simulink subsystem "s4EMSSC"  (R2024b)
settings: Solver=VariableStepAuto  StartTime=0.0  StopTime=10.0  RelTol=1e-3
undefined symbols (not defined in the file): EM1, EM2, EM3, EM4, HVDCNeg, HVDCPos, ThrmEM1, ThrmEM2, ThrmEM3, ThrmEM4
libraries: fl_lib x28, nesl_utility_internal x20
settings Model: ModifiedByFormat=The MathWorks, Inc.  Creator=The MathWorks, Inc.  LastModifiedBy=The MathWorks, Inc.
settings RTWCC: GPUComputeCapability=3.5

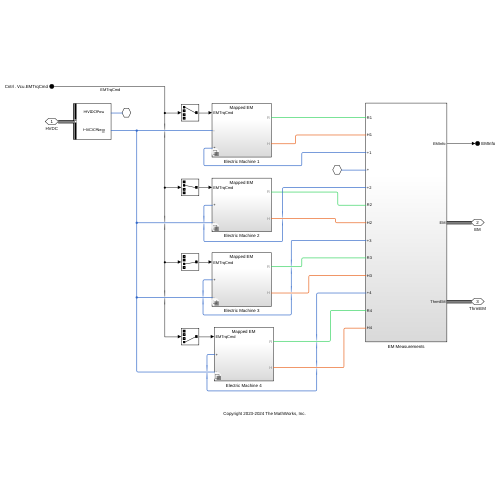
[thumbnail: Simulink's stored preview of the top-level diagram]
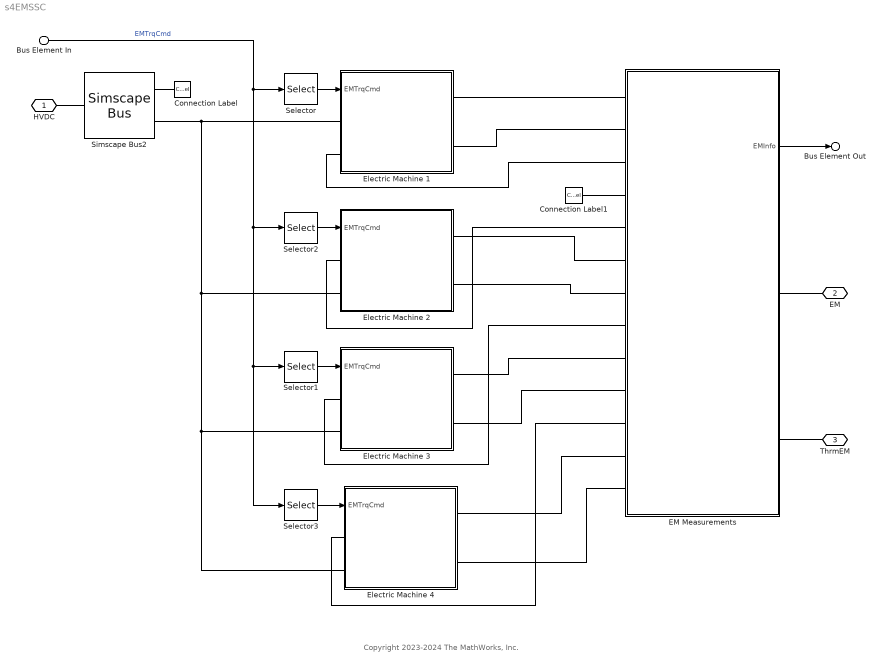
== system s4EMSSC ==
  note: Copyright 2023-2024 The MathWorks, Inc.
  Bus Element In : Inport  PortName=Cntrl  Element=Vcu.EMTrqCmd
  Connection Label : ConnectionLabel  Label=HVDCPos
  Connection Label1 : ConnectionLabel  Label=HVDCPos
  EM Measurements : Subsystem
  Electric Machine 1 : Subsystem  Variant=on  VariantControlMode=label  LabelModeActiveChoice=Mapped EM
  Electric Machine 2 : Subsystem  Variant=on  VariantControlMode=label  LabelModeActiveChoice=Mapped EM
  Electric Machine 3 : Subsystem  Variant=on  VariantControlMode=label  LabelModeActiveChoice=Mapped EM
  Electric Machine 4 : Subsystem  Variant=on  VariantControlMode=label  LabelModeActiveChoice=Mapped EM
  Selector : Selector  InputPortWidth=4  IndexOptions=Index vector (dialog)  Indices=[1]  OutputSizes=1
  Selector1 : Selector  InputPortWidth=4  IndexOptions=Index vector (dialog)  Indices=[3]  OutputSizes=1
  Selector2 : Selector  InputPortWidth=4  IndexOptions=Index vector (dialog)  Indices=[2]  OutputSizes=1
  Selector3 : Selector  InputPortWidth=4  IndexOptions=Index vector (dialog)  Indices=[4]  OutputSizes=1
  Simscape Bus2 : SimscapeBus  HierarchyStrings=HVDCPos;HVDCNeg
  HVDC : PMIOPort  Side=Left
  EM : PMIOPort  Port=2  Side=Right
  ThrmEM : PMIOPort  Port=3  Side=Right
  Bus Element Out : Outport  PortName=EMInfo
  wires:
  Selector3/1 -> Electric Machine 4/1(EMTrqCmd)
  Bus Element In/1 -> Selector2/1, Selector1/1, Selector3/1, Selector/1  "EMTrqCmd"
  Selector2/1 -> Electric Machine 2/1(EMTrqCmd)
  Selector/1 -> Electric Machine 1/1(EMTrqCmd)
  Selector1/1 -> Electric Machine 3/1(EMTrqCmd)
  EM Measurements/1(EMInfo) -> Bus Element Out/1
  connections:
  Simscape Bus2/LConn2 -- Electric Machine 3/LConn2 -- Electric Machine 4/LConn2 -- Electric Machine 2/LConn2 -- Electric Machine 1/LConn1
  HVDC/RConn1 -- Simscape Bus2/RConn1
  ThrmEM/RConn1 -- EM Measurements/RConn2
  EM Measurements/LConn9 -- Electric Machine 3/RConn1
  EM Measurements/LConn2 -- Electric Machine 1/RConn2
  EM Measurements/RConn1 -- EM/RConn1
  Electric Machine 2/RConn1 -- EM Measurements/LConn6
  Electric Machine 2/RConn2 -- EM Measurements/LConn7
  Electric Machine 1/RConn1 -- EM Measurements/LConn1
  EM Measurements/LConn5 -- Electric Machine 2/LConn1
  Connection Label1/LConn1 -- EM Measurements/LConn4
  Connection Label/LConn1 -- Simscape Bus2/LConn1
  EM Measurements/LConn3 -- Electric Machine 1/LConn2
  Electric Machine 3/LConn1 -- EM Measurements/LConn8
  Electric Machine 3/RConn2 -- EM Measurements/LConn10
  Electric Machine 4/LConn1 -- EM Measurements/LConn11
  Electric Machine 4/RConn1 -- EM Measurements/LConn12
  Electric Machine 4/RConn2 -- EM Measurements/LConn13

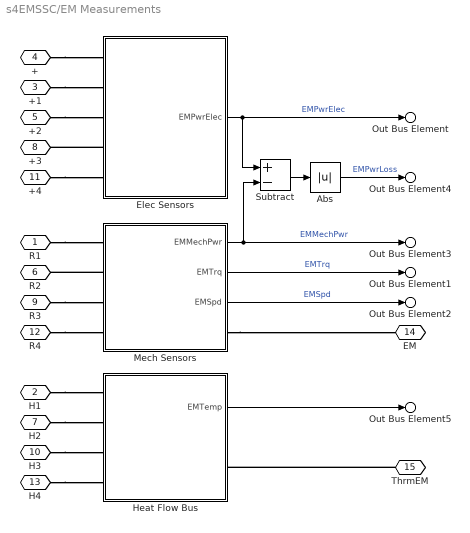
== system s4EMSSC/EM Measurements ==
  Abs : Abs  SaturateOnIntegerOverflow=off
  Elec Sensors : Subsystem
  Heat Flow Bus : Subsystem
  Mech Sensors : Subsystem
  Subtract : Sum  Inputs=+-
  R1 : PMIOPort  Side=Left
  H1 : PMIOPort  Port=2  Side=Left
  +1 : PMIOPort  Port=3  Side=Left
  + : PMIOPort  Port=4  Side=Left
  +2 : PMIOPort  Port=5  Side=Left
  R2 : PMIOPort  Port=6  Side=Left
  H2 : PMIOPort  Port=7  Side=Left
  +3 : PMIOPort  Port=8  Side=Left
  R3 : PMIOPort  Port=9  Side=Left
  H3 : PMIOPort  Port=10  Side=Left
  +4 : PMIOPort  Port=11  Side=Left
  R4 : PMIOPort  Port=12  Side=Left
  H4 : PMIOPort  Port=13  Side=Left
  EM : PMIOPort  Port=14  Side=Right
  ThrmEM : PMIOPort  Port=15  Side=Right
  Out Bus Element : Outport  PortName=EMInfo  Element=EMPwrElec
  Out Bus Element1 : Outport  PortName=EMInfo  Element=EMTrq
  Out Bus Element2 : Outport  PortName=EMInfo  Element=EMSpd
  Out Bus Element3 : Outport  PortName=EMInfo  Element=EMMechPwr
  Out Bus Element4 : Outport  PortName=EMInfo  Element=EMPwrLoss
  Out Bus Element5 : Outport  PortName=EMInfo  Element=EMTemp
  wires:
  Mech Sensors/1(EMMechPwr) -> Subtract/2, Out Bus Element3/1  "EMMechPwr"
  Mech Sensors/3(EMSpd) -> Out Bus Element2/1  "EMSpd"
  Mech Sensors/2(EMTrq) -> Out Bus Element1/1  "EMTrq"
  Elec Sensors/1(EMPwrElec) -> Subtract/1, Out Bus Element/1  "EMPwrElec"
  Abs/1 -> Out Bus Element4/1  "EMPwrLoss"
  Subtract/1 -> Abs/1
  Heat Flow Bus/1(EMTemp) -> Out Bus Element5/1
  connections:
  +4/RConn1 -- Elec Sensors/LConn5
  R4/RConn1 -- Mech Sensors/LConn4
  Elec Sensors/LConn4 -- +3/RConn1
  R3/RConn1 -- Mech Sensors/LConn3
  +2/RConn1 -- Elec Sensors/LConn3
  Mech Sensors/LConn2 -- R2/RConn1
  +1/RConn1 -- Elec Sensors/LConn2
  +/RConn1 -- Elec Sensors/LConn1
  R1/RConn1 -- Mech Sensors/LConn1
  ThrmEM/RConn1 -- Heat Flow Bus/RConn1
  Mech Sensors/RConn1 -- EM/RConn1
  H1/RConn1 -- Heat Flow Bus/LConn1
  H2/RConn1 -- Heat Flow Bus/LConn2
  H3/RConn1 -- Heat Flow Bus/LConn3
  H4/RConn1 -- Heat Flow Bus/LConn4

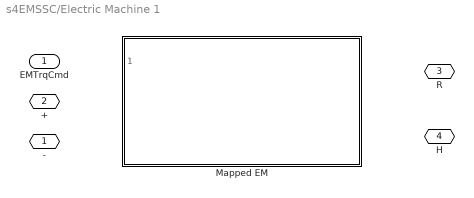
== system s4EMSSC/Electric Machine 1 ==
  EMTrqCmd : Inport
  Mapped EM : Subsystem  VariantControl=Mapped EM  ReferencedSubsystem=ElectricMachine1SSC
  - : PMIOPort  Side=Left
  + : PMIOPort  Port=2  Side=Left
  R : PMIOPort  Port=3  Side=Right
  H : PMIOPort  Port=4  Side=Right

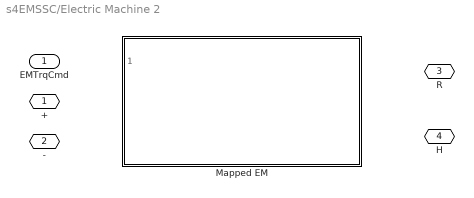
== system s4EMSSC/Electric Machine 2 ==
  EMTrqCmd : Inport
  Mapped EM : Subsystem  VariantControl=Mapped EM  ReferencedSubsystem=ElectricMachine2SSC
  + : PMIOPort  Side=Left
  - : PMIOPort  Port=2  Side=Left
  R : PMIOPort  Port=3  Side=Right
  H : PMIOPort  Port=4  Side=Right

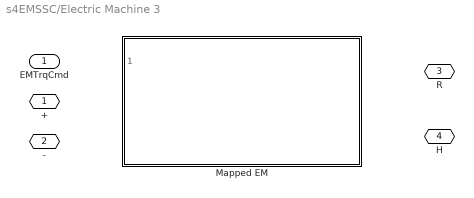
== system s4EMSSC/Electric Machine 3 ==
  EMTrqCmd : Inport
  Mapped EM : Subsystem  VariantControl=Mapped EM  ReferencedSubsystem=ElectricMachine3SSC
  + : PMIOPort  Side=Left
  - : PMIOPort  Port=2  Side=Left
  R : PMIOPort  Port=3  Side=Right
  H : PMIOPort  Port=4  Side=Right

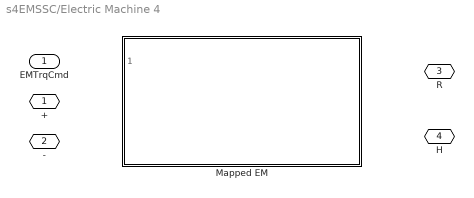
== system s4EMSSC/Electric Machine 4 ==
  EMTrqCmd : Inport
  Mapped EM : Subsystem  VariantControl=Mapped EM  ReferencedSubsystem=ElectricMachine4SSC
  + : PMIOPort  Side=Left
  - : PMIOPort  Port=2  Side=Left
  R : PMIOPort  Port=3  Side=Right
  H : PMIOPort  Port=4  Side=Right

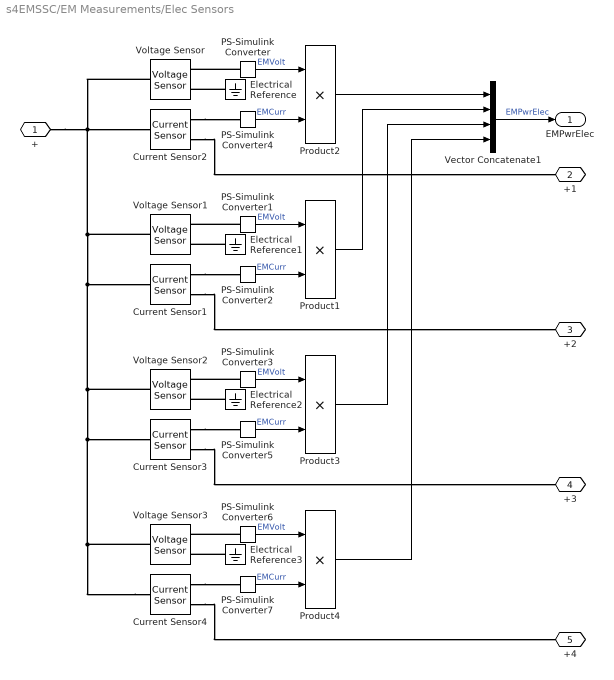
== system s4EMSSC/EM Measurements/Elec Sensors ==
  Current Sensor{1..4} (4 alike) : fl_lib/Electrical/Electrical Sensors/Current Sensor
  Electrical Reference{,1..3} (4 alike) : fl_lib/Electrical/Electrical Elements/Electrical Reference
  PS-Simulink Converter{,1,3,6} (4 alike) : nesl_utility_internal/PS-Simulink Converter  PhysicalDomain=network_engine_domain  SubClassName=ps_output  LeftPortType=input  RightPortType=output  PseudoPeriodic=off  Frequencies=[]  VectorFormat=1-D array  Unit=inherit  AffineConversion=off
  PS-Simulink Converter{2,4..5,7} (4 alike) : nesl_utility_internal/PS-Simulink Converter  PhysicalDomain=network_engine_domain  SubClassName=ps_output  LeftPortType=input  RightPortType=output  PseudoPeriodic=off  Frequencies=[]  VectorFormat=1-D array  Unit=1  AffineConversion=off
  Product{1..4} (4 alike) : Product
  Vector Concatenate1 : Concatenate  NumInputs=4
  Voltage Sensor{,1..3} (4 alike) : fl_lib/Electrical/Electrical Sensors/Voltage Sensor
  + : PMIOPort  Side=Left
  +1 : PMIOPort  Port=2  Side=Left
  +2 : PMIOPort  Port=3  Side=Left
  +3 : PMIOPort  Port=4  Side=Left
  +4 : PMIOPort  Port=5  Side=Left
  EMPwrElec : Outport
  wires:
  Product4/1 -> Vector Concatenate1/4
  PS-Simulink Converter7/1 -> Product4/2  "EMCurr"
  PS-Simulink Converter6/1 -> Product4/1  "EMVolt"
  PS-Simulink Converter3/1 -> Product3/1  "EMVolt"
  PS-Simulink Converter5/1 -> Product3/2  "EMCurr"
  Product3/1 -> Vector Concatenate1/3
  Product1/1 -> Vector Concatenate1/2
  Vector Concatenate1/1 -> EMPwrElec/1  "EMPwrElec"
  Product2/1 -> Vector Concatenate1/1
  PS-Simulink Converter2/1 -> Product1/2  "EMCurr"
  PS-Simulink Converter1/1 -> Product1/1  "EMVolt"
  PS-Simulink Converter/1 -> Product2/1  "EMVolt"
  PS-Simulink Converter4/1 -> Product2/2  "EMCurr"
  connections:
  Current Sensor4/RConn1 -- PS-Simulink Converter7/LConn1
  Current Sensor4/RConn2 -- +4/RConn1
  Electrical Reference3/LConn1 -- Voltage Sensor3/RConn2
  PS-Simulink Converter6/LConn1 -- Voltage Sensor3/RConn1
  PS-Simulink Converter3/LConn1 -- Voltage Sensor2/RConn1
  Electrical Reference2/LConn1 -- Voltage Sensor2/RConn2
  Current Sensor3/RConn2 -- +3/RConn1
  Current Sensor3/RConn1 -- PS-Simulink Converter5/LConn1
  Electrical Reference1/LConn1 -- Voltage Sensor1/RConn2
  Current Sensor1/RConn1 -- PS-Simulink Converter2/LConn1
  Current Sensor1/RConn2 -- +2/RConn1
  PS-Simulink Converter1/LConn1 -- Voltage Sensor1/RConn1
  PS-Simulink Converter/LConn1 -- Voltage Sensor/RConn1
  Electrical Reference/LConn1 -- Voltage Sensor/RConn2
  Current Sensor4/LConn1 -- Voltage Sensor3/LConn1 -- Voltage Sensor2/LConn1 -- Current Sensor2/LConn1 -- +/RConn1 -- Voltage Sensor/LConn1 -- Voltage Sensor1/LConn1 -- Current Sensor1/LConn1 -- Current Sensor3/LConn1
  Current Sensor2/RConn2 -- +1/RConn1
  Current Sensor2/RConn1 -- PS-Simulink Converter4/LConn1

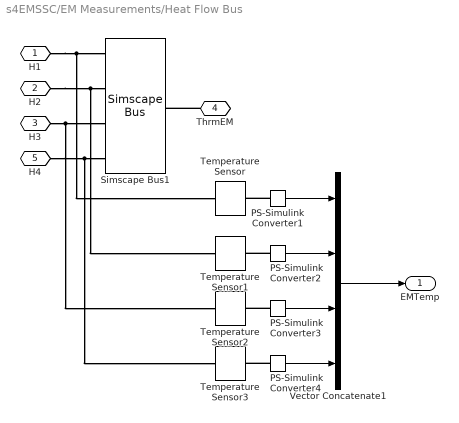
== system s4EMSSC/EM Measurements/Heat Flow Bus ==
  PS-Simulink Converter{1..4} (4 alike) : nesl_utility_internal/PS-Simulink Converter  PhysicalDomain=network_engine_domain  SubClassName=ps_output  LeftPortType=input  RightPortType=output  PseudoPeriodic=off  Frequencies=[]  VectorFormat=1-D array  Unit=K  AffineConversion=off
  Simscape Bus1 : SimscapeBus  HierarchyStrings=ThrmEM1;ThrmEM2;ThrmEM3;ThrmEM4
  Temperature Sensor{,1..3} (4 alike) : fl_lib/Thermal/Thermal Sensors/Temperature Sensor  temperature_measure=foundation.enum.MeasurementReference.absolute
      settings: InternalSimscapePortConfiguration="{\"Bottom\":[],\"Left\":[{\"id\":\"A\",\"label\":\"A\",\"type\":\"foundation.thermal.thermal\"}],\"Right\":[{\"id\":\"T\",\"label\":\"T\",\"type\":\"output\"}],\"Top\":[]}"
  Vector Concatenate1 : Concatenate  NumInputs=4
  H1 : PMIOPort  Side=Left
  H2 : PMIOPort  Port=2  Side=Left
  H3 : PMIOPort  Port=3  Side=Left
  ThrmEM : PMIOPort  Port=4  Side=Right
  H4 : PMIOPort  Port=5  Side=Left
  EMTemp : Outport
  wires:
  Vector Concatenate1/1 -> EMTemp/1
  PS-Simulink Converter3/1 -> Vector Concatenate1/3
  PS-Simulink Converter2/1 -> Vector Concatenate1/2
  PS-Simulink Converter1/1 -> Vector Concatenate1/1
  PS-Simulink Converter4/1 -> Vector Concatenate1/4
  connections:
  H1/RConn1 -- Temperature Sensor/LConn1 -- Simscape Bus1/LConn1
  H2/RConn1 -- Temperature Sensor1/LConn1 -- Simscape Bus1/LConn2
  H3/RConn1 -- Temperature Sensor2/LConn1 -- Simscape Bus1/LConn3
  ThrmEM/RConn1 -- Simscape Bus1/RConn1
  H4/RConn1 -- Temperature Sensor3/LConn1 -- Simscape Bus1/LConn4
  PS-Simulink Converter3/LConn1 -- Temperature Sensor2/RConn1
  PS-Simulink Converter2/LConn1 -- Temperature Sensor1/RConn1
  PS-Simulink Converter1/LConn1 -- Temperature Sensor/RConn1
  PS-Simulink Converter4/LConn1 -- Temperature Sensor3/RConn1

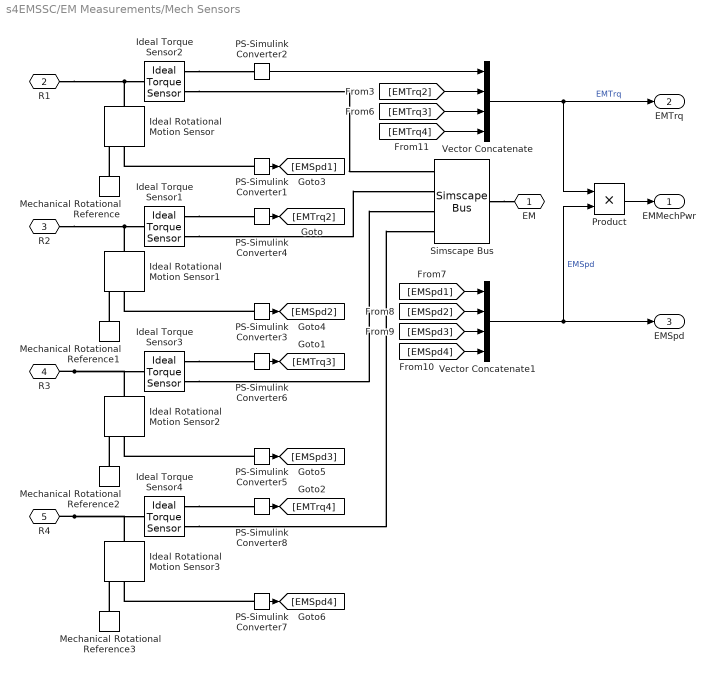
== system s4EMSSC/EM Measurements/Mech Sensors ==
  Ideal Rotational Motion Sensor{,1..3} (4 alike) : fl_lib/Mechanical/Mechanical Sensors/Ideal Rotational Motion Sensor  reference=foundation.enum.MeasurementReference.difference  acceleration_port=false  velocity_port=true  position_port=true  wrap_angle=false  offset=0 rad
  Ideal Torque Sensor{1..4} (4 alike) : fl_lib/Mechanical/Mechanical Sensors/Ideal Torque Sensor
  Mechanical Rotational Reference{,1..3} (4 alike) : fl_lib/Mechanical/Rotational Elements/Mechanical Rotational Reference
  PS-Simulink Converter{1,3,5,7} (4 alike) : nesl_utility_internal/PS-Simulink Converter  PhysicalDomain=network_engine_domain  SubClassName=ps_output  LeftPortType=input  RightPortType=output  PseudoPeriodic=off  Frequencies=[]  VectorFormat=1-D array  Unit=rad/s  AffineConversion=off
  PS-Simulink Converter{2,4,6,8} (4 alike) : nesl_utility_internal/PS-Simulink Converter  PhysicalDomain=network_engine_domain  SubClassName=ps_output  LeftPortType=input  RightPortType=output  PseudoPeriodic=off  Frequencies=[]  VectorFormat=1-D array  Unit=1  AffineConversion=off
  Product : Product
  Simscape Bus : SimscapeBus  HierarchyStrings=EM1;EM2;EM3;EM4
  Vector Concatenate : Concatenate  NumInputs=4
  Vector Concatenate1 : Concatenate  NumInputs=4
  EM : PMIOPort  Side=Right
  R1 : PMIOPort  Port=2  Side=Left
  R2 : PMIOPort  Port=3  Side=Left
  R3 : PMIOPort  Port=4  Side=Left
  R4 : PMIOPort  Port=5  Side=Left
  EMMechPwr : Outport
  EMTrq : Outport  Port=2
  EMSpd : Outport  Port=3
  wires:
  Product/1 -> EMMechPwr/1
  PS-Simulink Converter7/1 -> [EMSpd4]
  PS-Simulink Converter5/1 -> [EMSpd3]
  PS-Simulink Converter3/1 -> [EMSpd2]
  PS-Simulink Converter1/1 -> [EMSpd1]
  [EMSpd4] -> Vector Concatenate1/4
  [EMSpd3] -> Vector Concatenate1/3
  [EMSpd2] -> Vector Concatenate1/2
  [EMSpd1] -> Vector Concatenate1/1
  PS-Simulink Converter4/1 -> [EMTrq2]
  PS-Simulink Converter6/1 -> [EMTrq3]
  PS-Simulink Converter8/1 -> [EMTrq4]
  [EMTrq4] -> Vector Concatenate/4
  [EMTrq3] -> Vector Concatenate/3
  [EMTrq2] -> Vector Concatenate/2
  Vector Concatenate1/1 -> EMSpd/1, Product/2  "EMSpd"
  Vector Concatenate/1 -> EMTrq/1, Product/1  "EMTrq"
  PS-Simulink Converter2/1 -> Vector Concatenate/1
  connections:
  Ideal Torque Sensor4/RConn1 -- Simscape Bus/LConn4
  Mechanical Rotational Reference3/LConn1 -- Ideal Rotational Motion Sensor3/RConn1
  PS-Simulink Converter7/LConn1 -- Ideal Rotational Motion Sensor3/RConn2
  Ideal Torque Sensor4/RConn2 -- PS-Simulink Converter8/LConn1
  R4/RConn1 -- Ideal Rotational Motion Sensor3/LConn1 -- Ideal Torque Sensor4/LConn1
  Ideal Torque Sensor3/RConn2 -- PS-Simulink Converter6/LConn1
  Mechanical Rotational Reference2/LConn1 -- Ideal Rotational Motion Sensor2/RConn1
  Ideal Torque Sensor3/RConn1 -- Simscape Bus/LConn3
  PS-Simulink Converter5/LConn1 -- Ideal Rotational Motion Sensor2/RConn2
  R3/RConn1 -- Ideal Torque Sensor3/LConn1 -- Ideal Rotational Motion Sensor2/LConn1
  Simscape Bus/RConn1 -- EM/RConn1
  PS-Simulink Converter3/LConn1 -- Ideal Rotational Motion Sensor1/RConn2
  Ideal Torque Sensor1/RConn1 -- Simscape Bus/LConn2
  Mechanical Rotational Reference1/LConn1 -- Ideal Rotational Motion Sensor1/RConn1
  Ideal Torque Sensor1/RConn2 -- PS-Simulink Converter4/LConn1
  Ideal Rotational Motion Sensor1/LConn1 -- Ideal Torque Sensor1/LConn1 -- R2/RConn1
  PS-Simulink Converter1/LConn1 -- Ideal Rotational Motion Sensor/RConn2
  Mechanical Rotational Reference/LConn1 -- Ideal Rotational Motion Sensor/RConn1
  Ideal Torque Sensor2/RConn1 -- Simscape Bus/LConn1
  Ideal Rotational Motion Sensor/LConn1 -- R1/RConn1 -- Ideal Torque Sensor2/LConn1
  Ideal Torque Sensor2/RConn2 -- PS-Simulink Converter2/LConn1
